simulink model "MultirotorSimLin"  (R2017b)
settings: Solver=VariableStepAuto  StartTime=0.0  StopTime=Simulation.T_END  MaxStep=Simulation.TS_MAX  RelTol=1e-3  EnableMultiTasking=on
PreLoadFcn:
  | % InitializeParameters;
undefined symbols (not defined in the file): Initial
libraries: QuaternionLibrary x2, simulink_extras x1
settings Model: Creator=jban039  LastModifiedBy=jban039
settings DataIOCC: Decimation=10  ExternalInput=getinputstruct(op_trim3)  InitialState=getstatestruct(op_trim3)  ReturnWorkspaceOutputs=on  OutputOption=SpecifiedOutputTimes  OutputTimes=Simulation.T_OUT
settings OptimizationCC: LifeSpan=inf
settings DebuggingCC: ReadBeforeWriteMsg=DisableAll  WriteAfterWriteMsg=DisableAll  WriteAfterReadMsg=DisableAll  MultiTaskDSMMsg=none  UnconnectedLineMsg=none  AllowSymbolicDim=off  SFUnexpectedBacktrackingDiag=warning  SFNoUnconditionalDefaultTransitionDiag=warning  SFExecutionAtInitializationDiag=none
settings ModelReferenceCC: UpdateModelReferenceTargets=IfOutOfDate  ModelReferenceMinAlgLoopOccurrences=on  PropagateSignalLabelsOutOfModel=off
settings SFSimCC: SFSimEcho=off
settings CodeAppCC: StateflowObjectComments=on
settings GRTTargetCC: TargetLangStandard=C89/C90 (ANSI)
settings ConfigComp: CovMetricSettings=dw  CovHtmlReporting=on  CovSaveCumulativeToWorkspaceVar=on  CovSaveSingleToWorkspaceVar=on  CovExternalEMLEnable=off

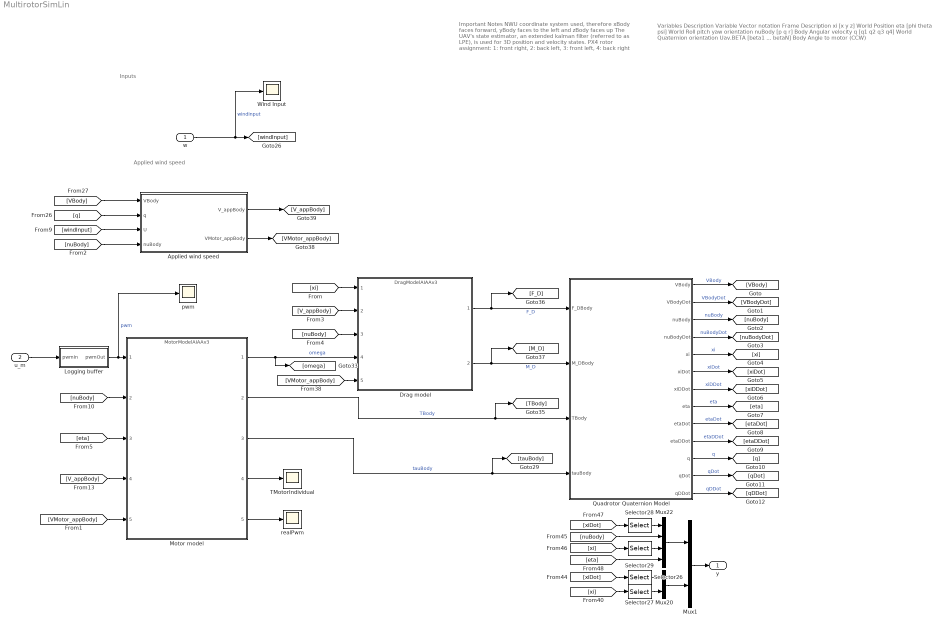
== system MultirotorSimLin ==
  note: Important Notes
      |
      | NWU coordinate system used, therefore xBody faces forward, yBody faces to the left and zBody faces up
      | The UAV's state estimator, an extended kalman filter (referred to as LPE), is used for 3D position and velocity states.
      | PX4 rotor assignment: 1: front right, 2: back left, 3: front left, 4: back right
  note: Variables Description
      |
      | Variable
      | Vector notation
      | Frame
      | Description
      |
      | xi
      | [x y z]
      | World
      | Position
      |
      | eta
      | [phi theta psi]
      | World
      | Roll pitch yaw orientation
      |
      | nuBody
      | [p q r]
      | Body
      | Angular velocity
      |
      | q
      | [q1 q2 q3 q4]
      | World
      | Quaternion orientation
      |
      | Uav.BETA
      | [beta1 ... betaN]
      | Body
      | Angle to motor (CCW)
  note: Applied wind speed
  note: Inputs
  w : Inport  PortDimensions=3
  u_m : Inport  Port=2  PortDimensions=4
  Applied wind speed : Subsystem
  Drag model : ModelReference  ModelNameDialog=DragModelAIAAv3  SimulationMode=Normal  ModelReferenceVersion=1.348
  Logging buffer : Subsystem
  Motor model : ModelReference  ModelNameDialog=MotorModelAIAAv3  SimulationMode=Normal  ModelReferenceVersion=1.358
  Mux1 : Mux  Inputs=2
  Mux20 : Mux  Inputs=2
  Mux22 : Mux
  Quadrotor Quaternion Model : Subsystem
  Selector26 : Selector  InputPortWidth=3  IndexOptions=Index vector (dialog)  Indices=[2 1]  OutputSizes=1
  Selector27 : Selector  InputPortWidth=3  IndexOptions=Index vector (dialog)  Indices=[2 1]  OutputSizes=1
  Selector28 : Selector  InputPortWidth=3  IndexOptions=Index vector (dialog)  Indices=3  OutputSizes=1
  Selector29 : Selector  InputPortWidth=3  IndexOptions=Index vector (dialog)  Indices=3  OutputSizes=1
  TMotorIndividual : Scope
  Wind Input : Scope
  pwm : Scope
  realPwm : Scope
  y : Outport
  wires:
  Motor model/1 -> [omega], Drag model/4  "omega"
  Motor model/2 -> Quadrotor Quaternion Model/3(TBody), [TBody]  "TBody"
  Drag model/2 -> Quadrotor Quaternion Model/2(M_DBody), [M_D]  "M_D"
  Quadrotor Quaternion Model/1(VBody) -> [VBody]  "VBody"
  Quadrotor Quaternion Model/2(VBodyDot) -> [VBodyDot]  "VBodyDot"
  Quadrotor Quaternion Model/3(nuBody) -> [nuBody]  "nuBody"
  Quadrotor Quaternion Model/4(nuBodyDot) -> [nuBodyDot]  "nuBodyDot"
  Quadrotor Quaternion Model/5(xi) -> [xi]  "xi"
  Quadrotor Quaternion Model/6(xiDot) -> [xiDot]  "xiDot"
  Quadrotor Quaternion Model/7(xiDDot) -> [xiDDot]  "xiDDot"
  Quadrotor Quaternion Model/8(eta) -> [eta]  "eta"
  Quadrotor Quaternion Model/9(etaDot) -> [etaDot]  "etaDot"
  Quadrotor Quaternion Model/10(etaDDot) -> [etaDDot]  "etaDDot"
  [V_appBody] -> Drag model/2
  [nuBody] -> Motor model/2
  Quadrotor Quaternion Model/11(q) -> [q]  "q"
  Quadrotor Quaternion Model/12(qDot) -> [qDot]  "qDot"
  Quadrotor Quaternion Model/13(qDDot) -> [qDDot]  "qDDot"
  Drag model/1 -> Quadrotor Quaternion Model/1(F_DBody), [F_D]  "F_D"
  Logging buffer/1(pwmOut) -> pwm/1, Motor model/1  "pwm"
  [nuBody] -> Drag model/3
  [eta] -> Motor model/3
  w/1 -> [windInput], Wind Input/1  "windInput"
  [V_appBody] -> Motor model/4
  Motor model/4 -> TMotorIndividual/1
  Motor model/5 -> realPwm/1
  [xi] -> Drag model/1
  [VMotor_appBody] -> Motor model/5
  [VMotor_appBody] -> Drag model/5
  Motor model/3 -> Quadrotor Quaternion Model/4(tauBody), [tauBody]  "tauBody"
  [VBody] -> Applied wind speed/1(VBody)
  [q] -> Applied wind speed/2(q)
  Applied wind speed/1(V_appBody) -> [V_appBody]
  Applied wind speed/2(VMotor_appBody) -> [VMotor_appBody]
  [nuBody] -> Applied wind speed/4(nuBody)
  [windInput] -> Applied wind speed/3(U)
  u_m/1 -> Logging buffer/1(pwmIn)
  Mux1/1 -> y/1
  Selector29/1 -> Mux22/3
  [xiDot] -> Selector28/1
  Selector28/1 -> Mux22/1
  [nuBody] -> Mux22/2
  Selector26/1 -> Mux20/1
  Selector27/1 -> Mux20/2
  [xi] -> Selector27/1
  [eta] -> Mux22/4
  [xi] -> Selector29/1
  [xiDot] -> Selector26/1
  Mux22/1 -> Mux1/1
  Mux20/1 -> Mux1/2

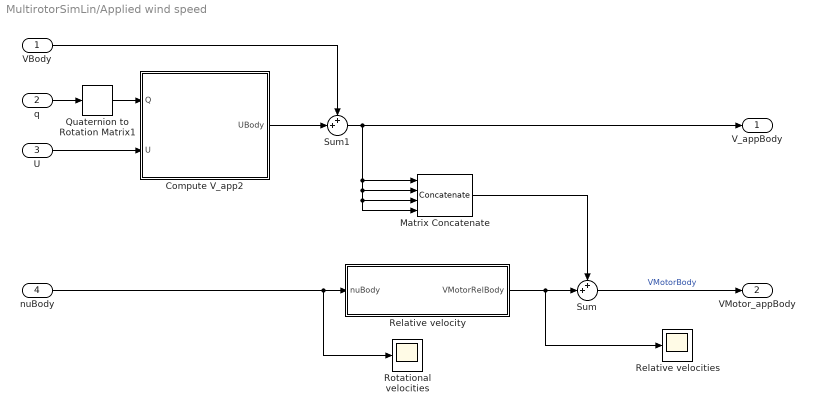
== system MultirotorSimLin/Applied wind speed ==
  VBody : Inport  Unit=m/s
  q : Inport  Port=2
  U : Inport  Port=3  Unit=m/s
  nuBody : Inport  Port=4  Unit=rad/s
  Compute V_app2 : MATLAB Function  TreatAsAtomicUnit=on
  Matrix Concatenate : Concatenate  NumInputs=4  Mode=Multidimensional array  ConcatenateDimension=2
  Quaternion to Rotation Matrix1 : QuaternionLibrary/Quaternion to Rotation Matrix
  Relative velocities : Scope
  Relative velocity : MATLAB Function  TreatAsAtomicUnit=on
  Rotational velocities : Scope
  Sum : Sum  Inputs=++|
  Sum1 : Sum  Inputs=++|
  V_appBody : Outport  Unit=m/s
  VMotor_appBody : Outport  Port=2  Unit=m/s
  wires:
  U/1 -> Compute V_app2/2(U)
  Sum/1 -> VMotor_appBody/1  "VMotorBody"
  Quaternion to Rotation Matrix1/1 -> Compute V_app2/1(Q)
  nuBody/1 -> Rotational velocities/1, Relative velocity/1(nuBody)
  Matrix Concatenate/1 -> Sum/1
  VBody/1 -> Sum1/1
  q/1 -> Quaternion to Rotation Matrix1/1
  Relative velocity/1(VMotorRelBody) -> Relative velocities/1, Sum/2
  Compute V_app2/1(UBody) -> Sum1/2
  Sum1/1 -> V_appBody/1, Matrix Concatenate/4, Matrix Concatenate/3, Matrix Concatenate/2, Matrix Concatenate/1

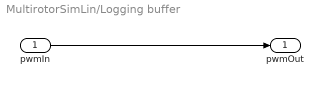
== system MultirotorSimLin/Logging buffer ==
  pwmIn : Inport
  pwmOut : Outport
  wires:
  pwmIn/1 -> pwmOut/1

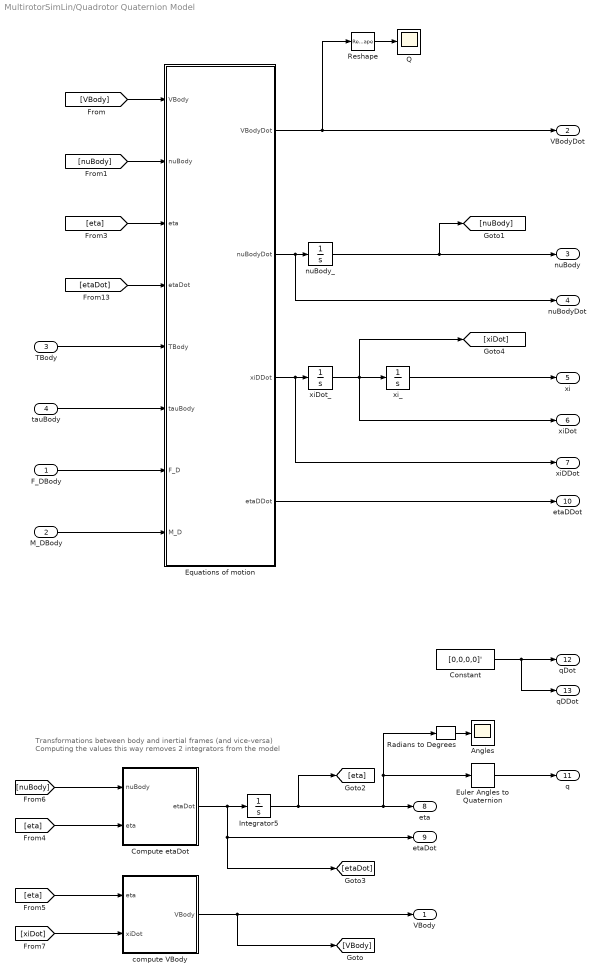
== system MultirotorSimLin/Quadrotor Quaternion Model ==
  note: Transformations between body and inertial frames (and vice-versa)
      | Computing the values this way removes 2 integrators from the model
  F_DBody : Inport  Unit=N
  M_DBody : Inport  Port=2  Unit=N*m
  TBody : Inport  Port=3  Unit=N
  tauBody : Inport  Port=4  Unit=N*m
  Angles : Scope
  Compute etaDot : MATLAB Function  TreatAsAtomicUnit=on
  Constant : Constant  Value=[0,0,0,0]'
  Equations of motion : MATLAB Function  TreatAsAtomicUnit=on
  Euler Angles to Quaternion : QuaternionLibrary/Euler Angles to Quaternion
  Integrator5 : Integrator  InitialCondition=Initial.ETA  ContinuousStateAttributes='eta'
  Q : Scope
  Radians to Degrees : simulink_extras/Transformations/Radians to Degrees
  Reshape : Reshape  OutputDimensionality=Column vector (2-D)
  compute VBody : MATLAB Function  TreatAsAtomicUnit=on
  nuBody_ : Integrator  InitialCondition=Initial.NU_BODY  ContinuousStateAttributes='nuBody'
  xiDot_ : Integrator  InitialCondition=Initial.XI_DOT  ContinuousStateAttributes='xiDot'
  xi_ : Integrator  InitialCondition=Initial.XI  ContinuousStateAttributes='xi'
  VBody : Outport  Unit=m/s
  VBodyDot : Outport  Port=2  Unit=m/s^2
  nuBody : Outport  Port=3  Unit=rad/s
  nuBodyDot : Outport  Port=4  Unit=rad/s^2
  xi : Outport  Port=5  Unit=m
  xiDot : Outport  Port=6  Unit=m/s
  xiDDot : Outport  Port=7  Unit=m/s^2
  eta : Outport  Port=8  Unit=rad
  etaDot : Outport  Port=9  Unit=rad/s
  etaDDot : Outport  Port=10  Unit=rad/s^2
  q : Outport  Port=11
  qDot : Outport  Port=12
  qDDot : Outport  Port=13
  wires:
  Equations of motion/1(VBodyDot) -> Reshape/1, VBodyDot/1
  xi_/1 -> xi/1
  [nuBody] -> Equations of motion/2(nuBody)
  [VBody] -> Equations of motion/1(VBody)
  tauBody/1 -> Equations of motion/6(tauBody)
  TBody/1 -> Equations of motion/5(TBody)
  Equations of motion/3(xiDDot) -> xiDot_/1, xiDDot/1
  F_DBody/1 -> Equations of motion/7(F_D)
  M_DBody/1 -> Equations of motion/8(M_D)
  nuBody_/1 -> [nuBody], nuBody/1
  Equations of motion/2(nuBodyDot) -> nuBody_/1, nuBodyDot/1
  [eta] -> Equations of motion/3(eta)
  Equations of motion/4(etaDDot) -> etaDDot/1
  Reshape/1 -> Q/1
  xiDot_/1 -> xi_/1, [xiDot], xiDot/1
  [etaDot] -> Equations of motion/4(etaDot)
  [xiDot] -> compute VBody/2(xiDot)
  [nuBody] -> Compute etaDot/1(nuBody)
  [eta] -> compute VBody/1(eta)
  compute VBody/1(VBody) -> VBody/1, [VBody]
  [eta] -> Compute etaDot/2(eta)
  Compute etaDot/1(etaDot) -> etaDot/1, [etaDot], Integrator5/1
  Integrator5/1 -> Radians to Degrees/1, Euler Angles to Quaternion/1, eta/1, [eta]
  Euler Angles to Quaternion/1 -> q/1
  Constant/1 -> qDDot/1, qDot/1
  Radians to Degrees/1 -> Angles/1

== matlab function MultirotorSimLin/Quadrotor Quaternion Model/Equations of motion ==
  data: VBody input; VBodyDot output; nuBody input; eta input; etaDot input; TBody input size=3; tauBody input size=3; F_D input size=3; M_D input size=3; nuBodyDot output; Uav parameter; xiDDot output; etaDDot output
function [VBodyDot, nuBodyDot, xiDDot, etaDDot] = QuadrotorQuaternionModel(...
    VBody, nuBody, eta, etaDot, TBody, tauBody, F_D, M_D, Uav )
%#codegen

%% Rotation matrices
% Precompute sines and cosines
sPhi   = sin(eta(1));
sTheta = sin(eta(2));
sPsi   = sin(eta(3));
cPhi   = cos(eta(1));
cTheta = cos(eta(2));
cPsi   = cos(eta(3));
tTheta = tan(eta(2));

phiDot   = etaDot(1);
thetaDot = etaDot(2);

% Body frame to inertial frame
R = [cPsi*cTheta, cPsi*sTheta*sPhi-sPsi*cPhi, cPsi*sTheta*cPhi+sPsi*sPhi;
     sPsi*cTheta, sPsi*sTheta*sPhi+cPsi*cPhi, sPsi*sTheta*cPhi-cPsi*sPhi;
     -sTheta,     cTheta*sPhi,                cTheta*cPhi+sPsi*sPhi];

WInvertDot = [...
    0,  phiDot*cPhi*tTheta+thetaDot*sPhi/cTheta^2,    -phiDot*sPhi*cTheta+thetaDot*cPhi/cTheta^2;
    0, -phiDot*sPhi,                                  -phiDot*cPhi;
	0,  phiDot*cPhi/cTheta+phiDot*sPhi*tTheta/cTheta, -phiDot*sPhi/cTheta+thetaDot*cPhi*tTheta/cTheta];

WInvert = [1, sPhi*tTheta,  cPhi*tTheta;
           0, cPhi,        -sPhi;
           0, sPhi/cTheta,  cPhi/cTheta];


%% Moments and Forces
% Body frame accelerations
VBodyDot  = (1/Uav.M) * (R'*Uav.G + TBody - cross(nuBody, Uav.M*VBody) + F_D);
nuBodyDot = Uav.I \ (tauBody - cross(nuBody, Uav.I*nuBody) + M_D);

% Inertial frame accelerations
xiDDot = (1/Uav.M)*(Uav.G + R*TBody + R*F_D);
etaDDot = WInvertDot*nuBody + WInvert*nuBodyDot;

end

== matlab function MultirotorSimLin/Applied wind speed/Relative velocity ==
  data: nuBody input; Uav parameter; VMotorRelBody output size=[3,4]
function VMotorRelBody = relativeMotorVelocity( nuBody , Uav )
%#codegen
assert(Uav.N_ROTORS < 16);

VMotorRelBody = zeros(3, 4);
% VMotorRelMotor = zeros(3, Uav.N_ROTORS);

for i = 1:length( Uav.N_ROTORS )
    VMotorRelBody(:,i) = cross( nuBody, Uav.L_VEC(:,i) );
    % VMotorRelMotor(:,i) = Uav.R_MOTOR_TO_BODY(:,:,i)' * VMotorRelBody;
end

== matlab function MultirotorSimLin/Applied wind speed/Compute V_app2 ==
  data: Q input; UBody output; U input size=3
function UBody = computeUBody(Q, U)
%#codegen

% Rotation matrix from Wind frame to Inertial frame 
R_U = [1, 0,  0;
       0, 1,  0;
       0, 0, -1];
   
UBody = Q' * R_U * U;

== matlab function MultirotorSimLin/Quadrotor Quaternion Model/Compute etaDot ==
  data: nuBody input; eta input; etaDot output
function etaDot = computeEtaDot(nuBody, eta)
%#codegen

sPhi = sin(eta(1));
cPhi = cos(eta(1));
cTheta = cos(eta(2));
tTheta = tan(eta(2));
      
WInverse = [1, sPhi*tTheta,  cPhi*tTheta;
            0, cPhi,        -sPhi;
            0, sPhi/cTheta,  cPhi/cTheta];

etaDot = WInverse*nuBody;

== matlab function MultirotorSimLin/Quadrotor Quaternion Model/compute VBody ==
  data: eta input; VBody output; xiDot input
function VBody = computeVBody(eta, xiDot)
%#codegen

sphi = sin(eta(1));
sTheta = sin(eta(2));
sPsi = sin(eta(3));
cPhi = cos(eta(1));
cTheta = cos(eta(2));
cPsi = cos(eta(3));

R = [ cPsi*cTheta, cPsi*sTheta*sphi-sPsi*cPhi, cPsi*sTheta*cPhi+sPsi*sphi;
	  sPsi*cTheta, sPsi*sTheta*sphi+cPsi*cPhi, sPsi*sTheta*cPhi-cPsi*sphi;
     -sTheta,      cTheta*sphi,                cTheta*cPhi+sPsi*sphi];

VBody = R'*xiDot;
